simulink model "TorqueControl"  (R2022a)
settings: Solver=VariableStepAuto  StartTime=0.0  StopTime=10.0  RelTol=1e-3
undefined symbols (not defined in the file): a, b, c, D, J, Kt, Tc
settings Model: Creator=sokse  LastModifiedBy=sokse

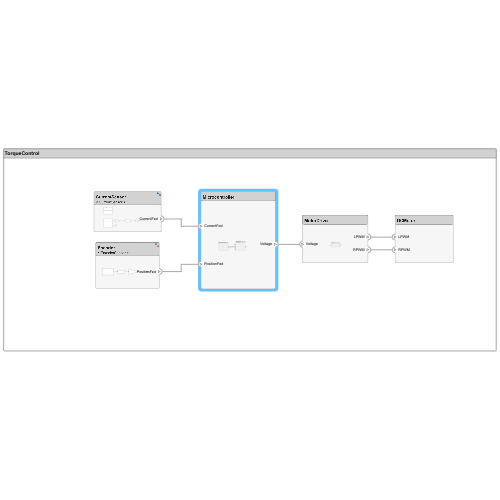
[thumbnail: Simulink's stored preview of the top-level diagram]
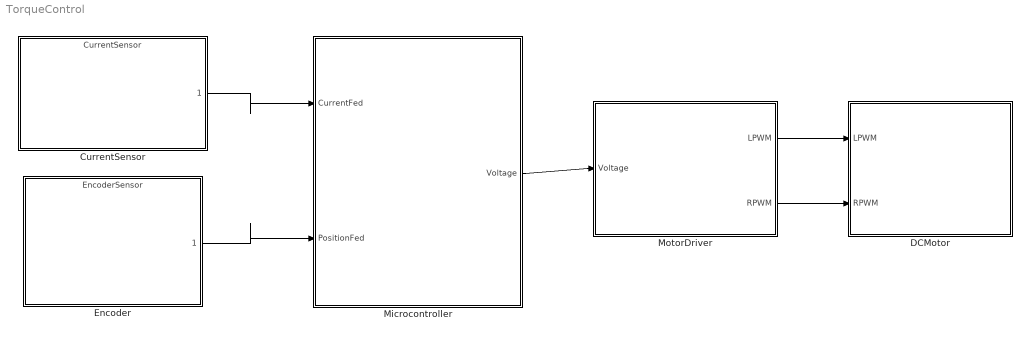
== system TorqueControl ==
  CurrentSensor : ModelReference  ModelNameDialog=CurrentSensor  SimulationMode=Normal  ModelReferenceVersion=1.3
      settings: PortSchema="{\"entries\":[{\"content\":{\"headerSize\":38,\"margin\":15,\"minimumSpacing\":25,\"sides\":[{\"content\":{\"connectorIds\":[]},\"type\":\"ConnectorPlacement.EquallySpacedRectSide\",\"uuid\":\"3b93c402-cac7-4c9a-af4f-66ab0cac09e6\"},{\"content\":{\"connectorIds\":[\"Out1\"],\"side\":\"RIGHT\"},\"type\":\"ConnectorPlacement.EquallySpacedRectSide\",\"uuid\":\"1c6ece9f-2b60-418c-8344-c12dccd361a4\"},{\"content\":{\"connectorIds\":[],\"side\":\"TOP\"},\"type\":\"ConnectorPlacement.EquallySpacedRectSide\",\"uuid\":\"b9a36c11-6150-4268-84cd-3d41a85e6a91\"}]},\"type\":\"ConnectorPlacement.EquallySpacedConnector\",\"uuid\":\"82b2256f-f535-4640-b6be-fef3a7c38360\"}],\"packageUris\":[\"http://schema.mathworks.com/mf0/Connector/R2020b\"],\"version\":\"1.0\"}"
  "DCMotor " : Subsystem
      settings: PortSchema="{\"entries\":[{\"content\":{\"headerSize\":26,\"margin\":15,\"minimumSpacing\":25,\"sides\":[{\"content\":{\"connectorIds\":[\"In2\",\"In1\"]},\"type\":\"ConnectorPlacement.EquallySpacedRectSide\",\"uuid\":\"3b93c402-cac7-4c9a-af4f-66ab0cac09e6\"},{\"content\":{\"connectorIds\":[],\"side\":\"RIGHT\"},\"type\":\"ConnectorPlacement.EquallySpacedRectSide\",\"uuid\":\"1c6ece9f-2b60-418c-8344-c12dccd361a4\"},{\"content\":{\"connectorIds\":[],\"side\":\"TOP\"},\"type\":\"ConnectorPlacement.EquallySpacedRectSide\",\"uuid\":\"b9a36c11-6150-4268-84cd-3d41a85e6a91\"},{\"content\":{\"connectorIds\":[],\"side\":\"BOTTOM\"},\"type\":\"ConnectorPlacement.EquallySpacedRectSide\",\"uuid\":\"e2681d5f-5760-4ff1-ab06-0e137d65a698\"}]},\"type\":\"ConnectorPlacement.EquallySpacedConnector\",\"uuid\":\"82b2256f-f535-4640-b6be-fef3a7c38360\"}],\"packageUris\":[\"http://schema.mathworks.com/mf0/Connector/R2020b\"],\"version\":\"1.0\"}"
  Encoder : ModelReference  ModelNameDialog=EncoderSensor  SimulationMode=Normal  ModelReferenceVersion=1.3
      settings: PortSchema="{\"entries\":[{\"content\":{\"headerSize\":38,\"margin\":15,\"minimumSpacing\":25,\"sides\":[{\"content\":{\"connectorIds\":[]},\"type\":\"ConnectorPlacement.EquallySpacedRectSide\",\"uuid\":\"3b93c402-cac7-4c9a-af4f-66ab0cac09e6\"},{\"content\":{\"connectorIds\":[\"Out1\"],\"side\":\"RIGHT\"},\"type\":\"ConnectorPlacement.EquallySpacedRectSide\",\"uuid\":\"1c6ece9f-2b60-418c-8344-c12dccd361a4\"},{\"content\":{\"connectorIds\":[],\"side\":\"TOP\"},\"type\":\"ConnectorPlacement.EquallySpacedRectSide\",\"uuid\":\"b9a36c11-6150-4268-84cd-3d41a85e6a91\"}]},\"type\":\"ConnectorPlacement.EquallySpacedConnector\",\"uuid\":\"82b2256f-f535-4640-b6be-fef3a7c38360\"}],\"packageUris\":[\"http://schema.mathworks.com/mf0/Connector/R2020b\"],\"version\":\"1.0\"}"
  Microcontroller : Subsystem
      settings: PortSchema="{\"entries\":[{\"content\":{\"headerSize\":26,\"margin\":15,\"minimumSpacing\":25,\"sides\":[{\"content\":{\"connectorIds\":[\"In1\",\"In2\"]},\"type\":\"ConnectorPlacement.EquallySpacedRectSide\",\"uuid\":\"3b93c402-cac7-4c9a-af4f-66ab0cac09e6\"},{\"content\":{\"connectorIds\":[\"Out1\"],\"side\":\"RIGHT\"},\"type\":\"ConnectorPlacement.EquallySpacedRectSide\",\"uuid\":\"1c6ece9f-2b60-418c-8344-c12dccd361a4\"},{\"content\":{\"connectorIds\":[],\"side\":\"TOP\"},\"type\":\"ConnectorPlacement.EquallySpacedRectSide\",\"uuid\":\"b9a36c11-6150-4268-84cd-3d41a85e6a91\"}]},\"type\":\"ConnectorPlacement.EquallySpacedConnector\",\"uuid\":\"82b2256f-f535-4640-b6be-fef3a7c38360\"}],\"packageUris\":[\"http://schema.mathworks.com/mf0/Connector/R2020b\"],\"version\":\"1.0\"}"
  MotorDriver : Subsystem
      settings: PortSchema="{\"entries\":[{\"content\":{\"headerSize\":26,\"margin\":15,\"minimumSpacing\":25,\"sides\":[{\"content\":{\"connectorIds\":[\"In1\"]},\"type\":\"ConnectorPlacement.EquallySpacedRectSide\",\"uuid\":\"3b93c402-cac7-4c9a-af4f-66ab0cac09e6\"},{\"content\":{\"connectorIds\":[\"Out1\",\"Out2\"],\"side\":\"RIGHT\"},\"type\":\"ConnectorPlacement.EquallySpacedRectSide\",\"uuid\":\"1c6ece9f-2b60-418c-8344-c12dccd361a4\"},{\"content\":{\"connectorIds\":[],\"side\":\"TOP\"},\"type\":\"ConnectorPlacement.EquallySpacedRectSide\",\"uuid\":\"b9a36c11-6150-4268-84cd-3d41a85e6a91\"}]},\"type\":\"ConnectorPlacement.EquallySpacedConnector\",\"uuid\":\"82b2256f-f535-4640-b6be-fef3a7c38360\"}],\"packageUris\":[\"http://schema.mathworks.com/mf0/Connector/R2020b\"],\"version\":\"1.0\"}"
  wires:
  Microcontroller/1(Voltage) -> MotorDriver/1(Voltage)
  MotorDriver/1(LPWM) -> "DCMotor "/2(LPWM)
  CurrentSensor/1 -> Microcontroller/1(CurrentFed)
  Encoder/1 -> Microcontroller/2(PositionFed)
  MotorDriver/2(RPWM) -> "DCMotor "/1(RPWM)

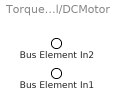
== system TorqueControl/DCMotor  ==
  Bus Element In1 : Inport  PortName=RPWM
  Bus Element In2 : Inport  Port=2  PortName=LPWM

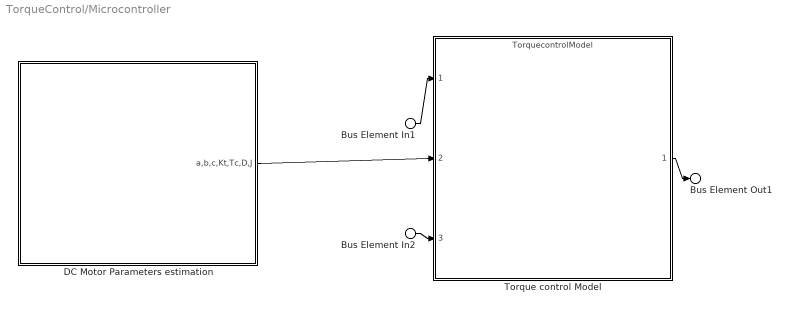
== system TorqueControl/Microcontroller ==
  Bus Element In1 : Inport  PortName=CurrentFed
  Bus Element In2 : Inport  Port=2  PortName=PositionFed
  "DC Motor Parameters estimation " : Subsystem
      settings: PortSchema="{\"entries\":[{\"content\":{\"headerSize\":26,\"margin\":15,\"minimumSpacing\":25,\"sides\":[{\"content\":{\"connectorIds\":[]},\"type\":\"ConnectorPlacement.EquallySpacedRectSide\",\"uuid\":\"3b93c402-cac7-4c9a-af4f-66ab0cac09e6\"},{\"content\":{\"connectorIds\":[\"Out1\"],\"side\":\"RIGHT\"},\"type\":\"ConnectorPlacement.EquallySpacedRectSide\",\"uuid\":\"1c6ece9f-2b60-418c-8344-c12dccd361a4\"},{\"content\":{\"connectorIds\":[],\"side\":\"TOP\"},\"type\":\"ConnectorPlacement.EquallySpacedRectSide\",\"uuid\":\"b9a36c11-6150-4268-84cd-3d41a85e6a91\"}]},\"type\":\"ConnectorPlacement.EquallySpacedConnector\",\"uuid\":\"82b2256f-f535-4640-b6be-fef3a7c38360\"}],\"packageUris\":[\"http://schema.mathworks.com/mf0/Connector/R2020b\"],\"version\":\"1.0\"}"
  "Torque control Model " : ModelReference  ModelNameDialog=TorquecontrolModel  SimulationMode=Normal  ModelReferenceVersion=1.3
      settings: PortSchema="{\"entries\":[{\"content\":{\"headerSize\":38,\"margin\":15,\"minimumSpacing\":25,\"sides\":[{\"content\":{\"connectorIds\":[\"In1\",\"In2\",\"In3\"]},\"type\":\"ConnectorPlacement.EquallySpacedRectSide\",\"uuid\":\"3b93c402-cac7-4c9a-af4f-66ab0cac09e6\"},{\"content\":{\"connectorIds\":[\"Out1\"],\"side\":\"RIGHT\"},\"type\":\"ConnectorPlacement.EquallySpacedRectSide\",\"uuid\":\"1c6ece9f-2b60-418c-8344-c12dccd361a4\"},{\"content\":{\"connectorIds\":[],\"side\":\"TOP\"},\"type\":\"ConnectorPlacement.EquallySpacedRectSide\",\"uuid\":\"b9a36c11-6150-4268-84cd-3d41a85e6a91\"}]},\"type\":\"ConnectorPlacement.EquallySpacedConnector\",\"uuid\":\"82b2256f-f535-4640-b6be-fef3a7c38360\"}],\"packageUris\":[\"http://schema.mathworks.com/mf0/Connector/R2020b\"],\"version\":\"1.0\"}"
  Bus Element Out1 : Outport  PortName=Voltage
  wires:
  Bus Element In1/1 -> "Torque control Model "/1
  Bus Element In2/1 -> "Torque control Model "/3
  "DC Motor Parameters estimation "/1(a,b,c,Kt,Tc,D,J) -> "Torque control Model "/2
  "Torque control Model "/1 -> Bus Element Out1/1

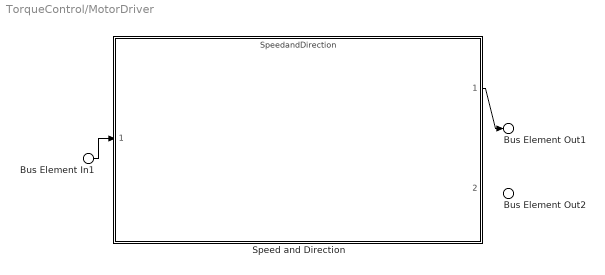
== system TorqueControl/MotorDriver ==
  Bus Element In1 : Inport  PortName=Voltage
  "Speed and Direction " : ModelReference  ModelNameDialog=SpeedandDirection  SimulationMode=Normal  ModelReferenceVersion=1.4
      settings: PortSchema="{\"entries\":[{\"content\":{\"headerSize\":38,\"margin\":15,\"minimumSpacing\":25,\"sides\":[{\"content\":{\"connectorIds\":[\"In1\"]},\"type\":\"ConnectorPlacement.EquallySpacedRectSide\",\"uuid\":\"3b93c402-cac7-4c9a-af4f-66ab0cac09e6\"},{\"content\":{\"connectorIds\":[\"Out1\",\"Out2\"],\"side\":\"RIGHT\"},\"type\":\"ConnectorPlacement.EquallySpacedRectSide\",\"uuid\":\"1c6ece9f-2b60-418c-8344-c12dccd361a4\"},{\"content\":{\"connectorIds\":[],\"side\":\"TOP\"},\"type\":\"ConnectorPlacement.EquallySpacedRectSide\",\"uuid\":\"b9a36c11-6150-4268-84cd-3d41a85e6a91\"}]},\"type\":\"ConnectorPlacement.EquallySpacedConnector\",\"uuid\":\"82b2256f-f535-4640-b6be-fef3a7c38360\"}],\"packageUris\":[\"http://schema.mathworks.com/mf0/Connector/R2020b\"],\"version\":\"1.0\"}"
  Bus Element Out1 : Outport  PortName=LPWM
  Bus Element Out2 : Outport  Port=2  PortName=RPWM
  wires:
  Bus Element In1/1 -> "Speed and Direction "/1
  "Speed and Direction "/1 -> Bus Element Out1/1

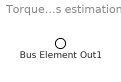
== system TorqueControl/Microcontroller/DC Motor Parameters estimation  ==
  Bus Element Out1 : Outport  PortName=a,b,c,Kt,Tc,D,J
